simulink model "IFSSIM_Drive"  (R2025b)
settings: Solver=ode1  StartTime=0  StopTime=8  FixedStep=1/960  RelTol=1e-3
undefined symbols (not defined in the file or in its folder): IFSSIM_EnvFlat, IFSSIM_RoadFlat, IFSSIM_SyncOff
settings Model: Creator=raulmoran  LastModifiedBy=raulmoran

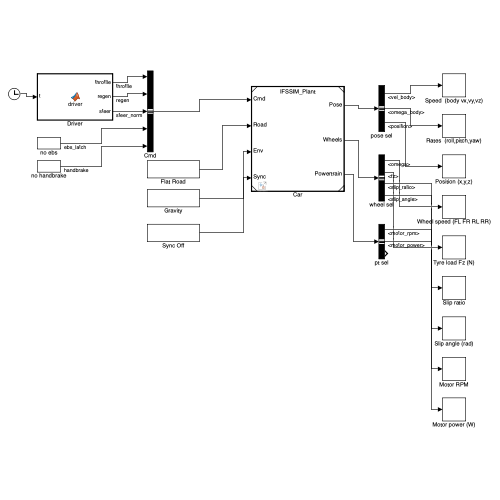
[thumbnail: Simulink's stored preview of the top-level diagram]
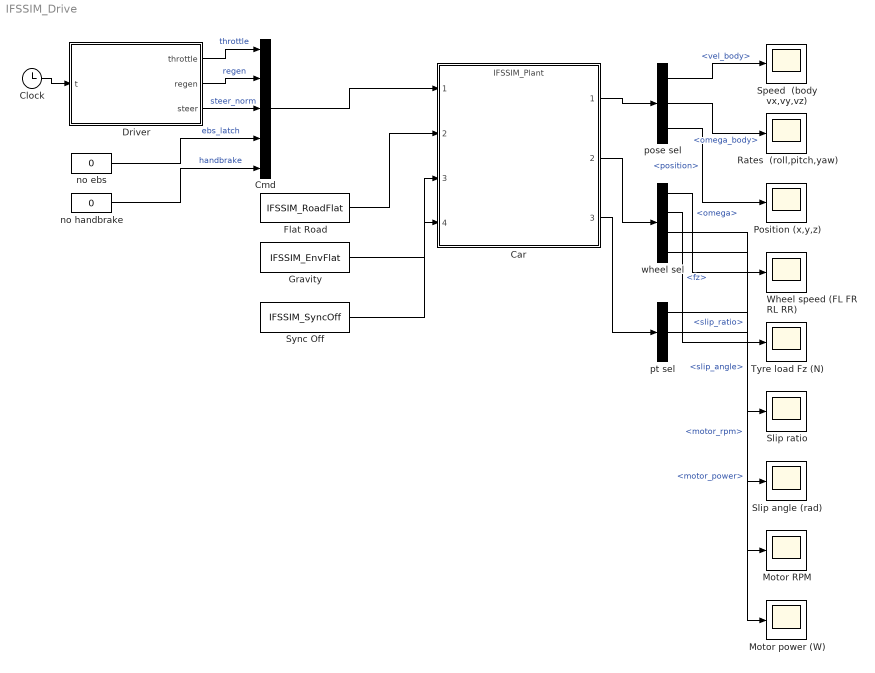
== system IFSSIM_Drive ==
  Car : ModelReference  ModelNameDialog=IFSSIM_Plant.slx  SimulationMode=Normal  ModelReferenceVersion=1.1
  Clock : Clock
  Cmd : BusCreator  Inputs=5  OutDataTypeStr=Bus: IFSSIM_CmdBus  NonVirtualBus=on
  Driver : MATLAB Function  TreatAsAtomicUnit=on
  Flat Road : Constant  Value=IFSSIM_RoadFlat  OutDataTypeStr=Bus: IFSSIM_RoadBus
  Gravity : Constant  Value=IFSSIM_EnvFlat  OutDataTypeStr=Bus: IFSSIM_EnvBus
  Motor RPM : Scope
  Motor power (W) : Scope
  Position (x,y,z) : Scope
  Rates  (roll,pitch,yaw) : Scope
  Slip angle (rad) : Scope
  Slip ratio : Scope
  Speed  (body vx,vy,vz) : Scope
  Sync Off : Constant  Value=IFSSIM_SyncOff  OutDataTypeStr=Bus: IFSSIM_SyncBus
  Tyre load Fz (N) : Scope
  Wheel speed (FL FR RL RR) : Scope
  no ebs : Constant  Value=0
  no handbrake : Constant  Value=0
  pose sel : BusSelector  OutputSignals=vel_body,omega_body,position
  pt sel : BusSelector  OutputSignals=motor_rpm,motor_power,batt_soc
  wheel sel : BusSelector  OutputSignals=omega,fz,slip_ratio,slip_angle
  wires:
  Clock/1 -> Driver/1(t)
  Driver/1(throttle) -> Cmd/1  "throttle"
  Driver/2(regen) -> Cmd/2  "regen"
  Driver/3(steer) -> Cmd/3  "steer_norm"
  no ebs/1 -> Cmd/4  "ebs_latch"
  no handbrake/1 -> Cmd/5  "handbrake"
  Cmd/1 -> Car/1
  Flat Road/1 -> Car/2
  Gravity/1 -> Car/3
  Sync Off/1 -> Car/4
  Car/1 -> pose sel/1
  Car/2 -> wheel sel/1
  Car/3 -> pt sel/1
  pose sel/1 -> Speed  (body vx,vy,vz)/1  "<vel_body>"
  pose sel/2 -> Rates  (roll,pitch,yaw)/1  "<omega_body>"
  pose sel/3 -> Position (x,y,z)/1  "<position>"
  wheel sel/1 -> Wheel speed (FL FR RL RR)/1  "<omega>"
  wheel sel/2 -> Tyre load Fz (N)/1  "<fz>"
  wheel sel/3 -> Slip ratio/1  "<slip_ratio>"
  wheel sel/4 -> Slip angle (rad)/1  "<slip_angle>"
  pt sel/1 -> Motor RPM/1  "<motor_rpm>"
  pt sel/2 -> Motor power (W)/1  "<motor_power>"

== matlab function IFSSIM_Drive/Driver ==
  data: t input size=1; throttle output size=1; regen output size=1; steer output size=1
function [throttle, regen, steer] = driver(t)
%#codegen
% The manoeuvre. Edit these four phases to change what the car does.
%
%   0-3 s   accelerate in a straight line
%   3-5 s   steady left turn, still on power
%   5-6 s   straighten and coast
%   6+  s   regen to a stop

throttle = 0; regen = 0; steer = 0;

if t < 3
    throttle = 0.5;
elseif t < 5
    throttle = 0.4;  steer = 0.4;
elseif t < 6
    throttle = 0.2;
else
    regen = 1.0;
end
end
